simulink library "speedgoatlib_bce"  (R2024b)
settings: Solver=VariableStepAuto  StartTime=0.0  StopTime=10.0  RelTol=1e-3
undefined symbols (not defined in the file): BCE12, BCE_Set_init, Cell_1, Cell_10, Cell_11, Cell_12, Cell_2, Cell_3, Cell_4, Cell_5, Cell_6, Cell_7, Cell_8, Cell_9, Device_01, FIU12, sg_bce, TSE04
libraries: slrealtimeethercatlib x292, simulink x92, slrealtimeutilitieslib x24
(part 3 of 4)

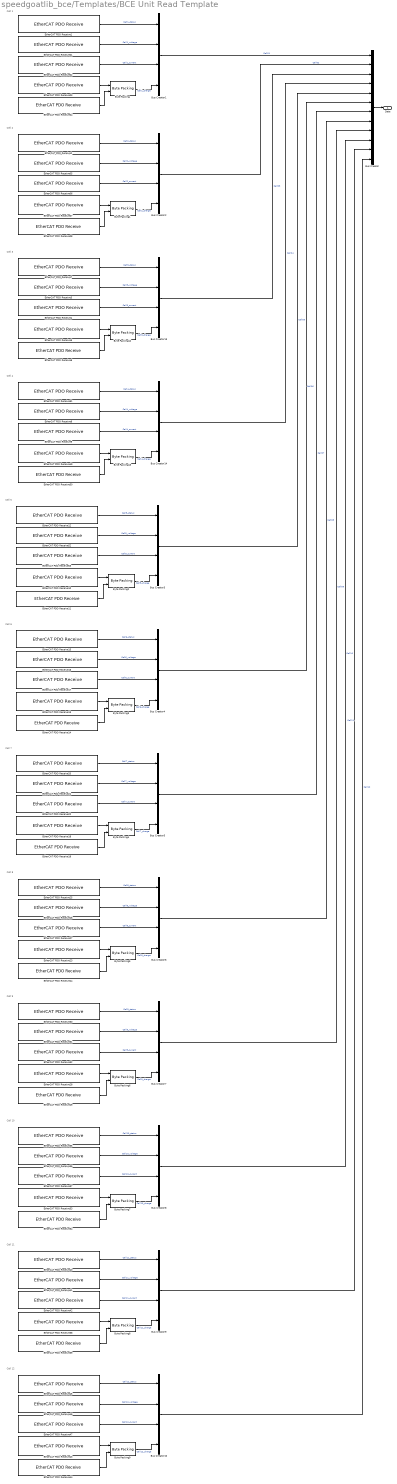
== system speedgoatlib_bce/Templates/BCE Unit Read Template  ==
  note: Cell 1
  note: Cell 9
  note: Cell 10
  note: Cell 4
  note: Cell 5
  note: Cell 3
  note: Cell 11
  note: Cell 12
  note: Cell 8
  note: Cell 6
  note: Cell 2
  note: Cell 7
  Bus Creator : BusCreator  Inputs=12  OutDataTypeStr=Bus: BCE_Get
      settings: InheritFromInputs=off
  Bus Creator{1..10,13..14} (12 alike) : BusCreator  Inputs=4  OutDataTypeStr=Bus: Cell_Get
      settings: InheritFromInputs=off
  Byte Packing{,1..9,12..13} (12 alike) : slrealtimeutilitieslib/Byte Packing  MaskPackedDataType=uint64  MaskUnpackedDataTypes={'uint32','uint32'}  MaskAlignment=1
  EtherCAT PDO Receive01 : slrealtimeethercatlib/EtherCAT PDO Receive  Priority=2  sig_name=Device_01 (BCE12-0505).Tx_Cell_01.voltage  sig_offset=16  sig_type=single  type_size=32  sig_dim=1  device_id=0  sample_time=0.000000
  EtherCAT PDO Receive02 : slrealtimeethercatlib/EtherCAT PDO Receive  Priority=2  sig_name=Device_01 (BCE12-0505).Tx_Cell_01.current  sig_offset=48  sig_type=single  type_size=32  sig_dim=1  device_id=0  sample_time=0.000000
  EtherCAT PDO Receive03 : slrealtimeethercatlib/EtherCAT PDO Receive  Priority=2  sig_name=Device_01 (BCE12-0505).Tx_Cell_01.chargeMSB  sig_offset=80  sig_type=uint32  type_size=32  sig_dim=1  device_id=0  sample_time=0.000000
  EtherCAT PDO Receive04 : slrealtimeethercatlib/EtherCAT PDO Receive  Priority=2  sig_name=Device_01 (BCE12-0505).Tx_Cell_01.chargeLSB  sig_offset=112  sig_type=uint32  type_size=32  sig_dim=1  device_id=0  sample_time=0.000000
  EtherCAT PDO Receive05 : slrealtimeethercatlib/EtherCAT PDO Receive  Priority=2  sig_name=Device_01 (BCE12-0505).Tx_Cell_02.voltage  sig_offset=160  sig_type=single  type_size=32  sig_dim=1  device_id=0  sample_time=0.000000
  EtherCAT PDO Receive06 : slrealtimeethercatlib/EtherCAT PDO Receive  Priority=2  sig_name=Device_01 (BCE12-0505).Tx_Cell_02.current  sig_offset=192  sig_type=single  type_size=32  sig_dim=1  device_id=0  sample_time=0.000000
  EtherCAT PDO Receive07 : slrealtimeethercatlib/EtherCAT PDO Receive  Priority=2  sig_name=Device_01 (BCE12-0505).Tx_Cell_02.chargeMSB  sig_offset=224  sig_type=uint32  type_size=32  sig_dim=1  device_id=0  sample_time=0.000000
  EtherCAT PDO Receive08 : slrealtimeethercatlib/EtherCAT PDO Receive  Priority=2  sig_name=Device_01 (BCE12-0505).Tx_Cell_02.chargeLSB  sig_offset=256  sig_type=uint32  type_size=32  sig_dim=1  device_id=0  sample_time=0.000000
  EtherCAT PDO Receive1 : slrealtimeethercatlib/EtherCAT PDO Receive  Priority=2  sig_name=Device_01 (BCE12-0505).Tx_Cell_01.status  sig_offset=0  sig_type=uint16  type_size=16  sig_dim=1  device_id=0  sample_time=0.000000
  EtherCAT PDO Receive10 : slrealtimeethercatlib/EtherCAT PDO Receive  Priority=2  sig_name=Device_01 (BCE12-0505).Tx_Cell_05.chargeMSB  sig_offset=656  sig_type=uint32  type_size=32  sig_dim=1  device_id=0  sample_time=0.000000
  EtherCAT PDO Receive11 : slrealtimeethercatlib/EtherCAT PDO Receive  Priority=2  sig_name=Device_01 (BCE12-0505).Tx_Cell_05.chargeLSB  sig_offset=688  sig_type=uint32  type_size=32  sig_dim=1  device_id=0  sample_time=0.000000
  EtherCAT PDO Receive12 : slrealtimeethercatlib/EtherCAT PDO Receive  Priority=2  sig_name=Device_01 (BCE12-0505).Tx_Cell_05.status  sig_offset=576  sig_type=uint16  type_size=16  sig_dim=1  device_id=0  sample_time=0.000000
  EtherCAT PDO Receive13 : slrealtimeethercatlib/EtherCAT PDO Receive  Priority=2  sig_name=Device_01 (BCE12-0505).Tx_Cell_06.chargeMSB  sig_offset=800  sig_type=uint32  type_size=32  sig_dim=1  device_id=0  sample_time=0.000000
  EtherCAT PDO Receive14 : slrealtimeethercatlib/EtherCAT PDO Receive  Priority=2  sig_name=Device_01 (BCE12-0505).Tx_Cell_06.chargeLSB  sig_offset=832  sig_type=uint32  type_size=32  sig_dim=1  device_id=0  sample_time=0.000000
  EtherCAT PDO Receive15 : slrealtimeethercatlib/EtherCAT PDO Receive  Priority=2  sig_name=Device_01 (BCE12-0505).Tx_Cell_06.status  sig_offset=720  sig_type=uint16  type_size=16  sig_dim=1  device_id=0  sample_time=0.000000
  EtherCAT PDO Receive16 : slrealtimeethercatlib/EtherCAT PDO Receive  Priority=2  sig_name=Device_01 (BCE12-0505).Tx_Cell_06.voltage  sig_offset=736  sig_type=single  type_size=32  sig_dim=1  device_id=0  sample_time=0.000000
  EtherCAT PDO Receive17 : slrealtimeethercatlib/EtherCAT PDO Receive  Priority=2  sig_name=Device_01 (BCE12-0505).Tx_Cell_06.current  sig_offset=768  sig_type=single  type_size=32  sig_dim=1  device_id=0  sample_time=0.000000
  EtherCAT PDO Receive18 : slrealtimeethercatlib/EtherCAT PDO Receive  Priority=2  sig_name=Device_01 (BCE12-0505).Tx_Cell_07.chargeMSB  sig_offset=944  sig_type=uint32  type_size=32  sig_dim=1  device_id=0  sample_time=0.000000
  EtherCAT PDO Receive19 : slrealtimeethercatlib/EtherCAT PDO Receive  Priority=2  sig_name=Device_01 (BCE12-0505).Tx_Cell_07.chargeLSB  sig_offset=976  sig_type=uint32  type_size=32  sig_dim=1  device_id=0  sample_time=0.000000
  EtherCAT PDO Receive2 : slrealtimeethercatlib/EtherCAT PDO Receive  Priority=2  sig_name=Device_01 (BCE12-0505).Tx_Cell_02.status  sig_offset=144  sig_type=uint16  type_size=16  sig_dim=1  device_id=0  sample_time=0.000000
  EtherCAT PDO Receive20 : slrealtimeethercatlib/EtherCAT PDO Receive  Priority=2  sig_name=Device_01 (BCE12-0505).Tx_Cell_07.status  sig_offset=864  sig_type=uint16  type_size=16  sig_dim=1  device_id=0  sample_time=0.000000
  EtherCAT PDO Receive21 : slrealtimeethercatlib/EtherCAT PDO Receive  Priority=2  sig_name=Device_01 (BCE12-0505).Tx_Cell_07.voltage  sig_offset=880  sig_type=single  type_size=32  sig_dim=1  device_id=0  sample_time=0.000000
  EtherCAT PDO Receive22 : slrealtimeethercatlib/EtherCAT PDO Receive  Priority=2  sig_name=Device_01 (BCE12-0505).Tx_Cell_07.current  sig_offset=912  sig_type=single  type_size=32  sig_dim=1  device_id=0  sample_time=0.000000
  EtherCAT PDO Receive23 : slrealtimeethercatlib/EtherCAT PDO Receive  Priority=2  sig_name=Device_01 (BCE12-0505).Tx_Cell_08.chargeMSB  sig_offset=1088  sig_type=uint32  type_size=32  sig_dim=1  device_id=0  sample_time=0.000000
  EtherCAT PDO Receive24 : slrealtimeethercatlib/EtherCAT PDO Receive  Priority=2  sig_name=Device_01 (BCE12-0505).Tx_Cell_08.chargeLSB  sig_offset=1120  sig_type=uint32  type_size=32  sig_dim=1  device_id=0  sample_time=0.000000
  EtherCAT PDO Receive25 : slrealtimeethercatlib/EtherCAT PDO Receive  Priority=2  sig_name=Device_01 (BCE12-0505).Tx_Cell_08.status  sig_offset=1008  sig_type=uint16  type_size=16  sig_dim=1  device_id=0  sample_time=0.000000
  EtherCAT PDO Receive26 : slrealtimeethercatlib/EtherCAT PDO Receive  Priority=2  sig_name=Device_01 (BCE12-0505).Tx_Cell_08.voltage  sig_offset=1024  sig_type=single  type_size=32  sig_dim=1  device_id=0  sample_time=0.000000
  EtherCAT PDO Receive27 : slrealtimeethercatlib/EtherCAT PDO Receive  Priority=2  sig_name=Device_01 (BCE12-0505).Tx_Cell_08.current  sig_offset=1056  sig_type=single  type_size=32  sig_dim=1  device_id=0  sample_time=0.000000
  EtherCAT PDO Receive28 : slrealtimeethercatlib/EtherCAT PDO Receive  Priority=2  sig_name=Device_01 (BCE12-0505).Tx_Cell_09.chargeMSB  sig_offset=1232  sig_type=uint32  type_size=32  sig_dim=1  device_id=0  sample_time=0.000000
  EtherCAT PDO Receive29 : slrealtimeethercatlib/EtherCAT PDO Receive  Priority=2  sig_name=Device_01 (BCE12-0505).Tx_Cell_09.chargeLSB  sig_offset=1264  sig_type=uint32  type_size=32  sig_dim=1  device_id=0  sample_time=0.000000
  EtherCAT PDO Receive3 : slrealtimeethercatlib/EtherCAT PDO Receive  Priority=2  sig_name=Device_01 (BCE12-0505).Tx_Cell_03.voltage  sig_offset=304  sig_type=single  type_size=32  sig_dim=1  device_id=0  sample_time=0.000000
  EtherCAT PDO Receive30 : slrealtimeethercatlib/EtherCAT PDO Receive  Priority=2  sig_name=Device_01 (BCE12-0505).Tx_Cell_09.status  sig_offset=1152  sig_type=uint16  type_size=16  sig_dim=1  device_id=0  sample_time=0.000000
  EtherCAT PDO Receive31 : slrealtimeethercatlib/EtherCAT PDO Receive  Priority=2  sig_name=Device_01 (BCE12-0505).Tx_Cell_09.voltage  sig_offset=1168  sig_type=single  type_size=32  sig_dim=1  device_id=0  sample_time=0.000000
  EtherCAT PDO Receive32 : slrealtimeethercatlib/EtherCAT PDO Receive  Priority=2  sig_name=Device_01 (BCE12-0505).Tx_Cell_09.current  sig_offset=1200  sig_type=single  type_size=32  sig_dim=1  device_id=0  sample_time=0.000000
  EtherCAT PDO Receive33 : slrealtimeethercatlib/EtherCAT PDO Receive  Priority=2  sig_name=Device_01 (BCE12-0505).Tx_Cell_10.chargeMSB  sig_offset=1376  sig_type=uint32  type_size=32  sig_dim=1  device_id=0  sample_time=0.000000
  EtherCAT PDO Receive34 : slrealtimeethercatlib/EtherCAT PDO Receive  Priority=2  sig_name=Device_01 (BCE12-0505).Tx_Cell_10.chargeLSB  sig_offset=1408  sig_type=uint32  type_size=32  sig_dim=1  device_id=0  sample_time=0.000000
  EtherCAT PDO Receive35 : slrealtimeethercatlib/EtherCAT PDO Receive  Priority=2  sig_name=Device_01 (BCE12-0505).Tx_Cell_10.status  sig_offset=1296  sig_type=uint16  type_size=16  sig_dim=1  device_id=0  sample_time=0.000000
  EtherCAT PDO Receive36 : slrealtimeethercatlib/EtherCAT PDO Receive  Priority=2  sig_name=Device_01 (BCE12-0505).Tx_Cell_10.voltage  sig_offset=1312  sig_type=single  type_size=32  sig_dim=1  device_id=0  sample_time=0.000000
  EtherCAT PDO Receive37 : slrealtimeethercatlib/EtherCAT PDO Receive  Priority=2  sig_name=Device_01 (BCE12-0505).Tx_Cell_10.current  sig_offset=1344  sig_type=single  type_size=32  sig_dim=1  device_id=0  sample_time=0.000000
  EtherCAT PDO Receive38 : slrealtimeethercatlib/EtherCAT PDO Receive  Priority=2  sig_name=Device_01 (BCE12-0505).Tx_Cell_11.chargeMSB  sig_offset=1520  sig_type=uint32  type_size=32  sig_dim=1  device_id=0  sample_time=0.000000
  EtherCAT PDO Receive39 : slrealtimeethercatlib/EtherCAT PDO Receive  Priority=2  sig_name=Device_01 (BCE12-0505).Tx_Cell_11.chargeLSB  sig_offset=1552  sig_type=uint32  type_size=32  sig_dim=1  device_id=0  sample_time=0.000000
  EtherCAT PDO Receive4 : slrealtimeethercatlib/EtherCAT PDO Receive  Priority=2  sig_name=Device_01 (BCE12-0505).Tx_Cell_03.current  sig_offset=336  sig_type=single  type_size=32  sig_dim=1  device_id=0  sample_time=0.000000
  EtherCAT PDO Receive40 : slrealtimeethercatlib/EtherCAT PDO Receive  Priority=2  sig_name=Device_01 (BCE12-0505).Tx_Cell_11.status  sig_offset=1440  sig_type=uint16  type_size=16  sig_dim=1  device_id=0  sample_time=0.000000
  EtherCAT PDO Receive41 : slrealtimeethercatlib/EtherCAT PDO Receive  Priority=2  sig_name=Device_01 (BCE12-0505).Tx_Cell_11.voltage  sig_offset=1456  sig_type=single  type_size=32  sig_dim=1  device_id=0  sample_time=0.000000
  EtherCAT PDO Receive42 : slrealtimeethercatlib/EtherCAT PDO Receive  Priority=2  sig_name=Device_01 (BCE12-0505).Tx_Cell_11.current  sig_offset=1488  sig_type=single  type_size=32  sig_dim=1  device_id=0  sample_time=0.000000
  EtherCAT PDO Receive43 : slrealtimeethercatlib/EtherCAT PDO Receive  Priority=2  sig_name=Device_01 (BCE12-0505).Tx_Cell_12.chargeMSB  sig_offset=1664  sig_type=uint32  type_size=32  sig_dim=1  device_id=0  sample_time=0.000000
  EtherCAT PDO Receive44 : slrealtimeethercatlib/EtherCAT PDO Receive  Priority=2  sig_name=Device_01 (BCE12-0505).Tx_Cell_12.chargeLSB  sig_offset=1696  sig_type=uint32  type_size=32  sig_dim=1  device_id=0  sample_time=0.000000
  EtherCAT PDO Receive45 : slrealtimeethercatlib/EtherCAT PDO Receive  Priority=2  sig_name=Device_01 (BCE12-0505).Tx_Cell_12.status  sig_offset=1584  sig_type=uint16  type_size=16  sig_dim=1  device_id=0  sample_time=0.000000
  EtherCAT PDO Receive46 : slrealtimeethercatlib/EtherCAT PDO Receive  Priority=2  sig_name=Device_01 (BCE12-0505).Tx_Cell_12.voltage  sig_offset=1600  sig_type=single  type_size=32  sig_dim=1  device_id=0  sample_time=0.000000
  EtherCAT PDO Receive47 : slrealtimeethercatlib/EtherCAT PDO Receive  Priority=2  sig_name=Device_01 (BCE12-0505).Tx_Cell_12.current  sig_offset=1632  sig_type=single  type_size=32  sig_dim=1  device_id=0  sample_time=0.000000
  EtherCAT PDO Receive49 : slrealtimeethercatlib/EtherCAT PDO Receive  Priority=2  sig_name=Device_01 (BCE12-0505).Tx_Cell_04.chargeMSB  sig_offset=512  sig_type=uint32  type_size=32  sig_dim=1  device_id=0  sample_time=0.000000
  EtherCAT PDO Receive5 : slrealtimeethercatlib/EtherCAT PDO Receive  Priority=2  sig_name=Device_01 (BCE12-0505).Tx_Cell_03.chargeMSB  sig_offset=368  sig_type=uint32  type_size=32  sig_dim=1  device_id=0  sample_time=0.000000
  EtherCAT PDO Receive50 : slrealtimeethercatlib/EtherCAT PDO Receive  Priority=2  sig_name=Device_01 (BCE12-0505).Tx_Cell_04.chargeLSB  sig_offset=544  sig_type=uint32  type_size=32  sig_dim=1  device_id=0  sample_time=0.000000
  EtherCAT PDO Receive51 : slrealtimeethercatlib/EtherCAT PDO Receive  Priority=2  sig_name=Device_01 (BCE12-0505).Tx_Cell_04.status  sig_offset=432  sig_type=uint16  type_size=16  sig_dim=1  device_id=0  sample_time=0.000000
  EtherCAT PDO Receive52 : slrealtimeethercatlib/EtherCAT PDO Receive  Priority=2  sig_name=Device_01 (BCE12-0505).Tx_Cell_05.voltage  sig_offset=592  sig_type=single  type_size=32  sig_dim=1  device_id=0  sample_time=0.000000
  EtherCAT PDO Receive53 : slrealtimeethercatlib/EtherCAT PDO Receive  Priority=2  sig_name=Device_01 (BCE12-0505).Tx_Cell_05.current  sig_offset=624  sig_type=single  type_size=32  sig_dim=1  device_id=0  sample_time=0.000000
  EtherCAT PDO Receive6 : slrealtimeethercatlib/EtherCAT PDO Receive  Priority=2  sig_name=Device_01 (BCE12-0505).Tx_Cell_03.chargeLSB  sig_offset=400  sig_type=uint32  type_size=32  sig_dim=1  device_id=0  sample_time=0.000000
  EtherCAT PDO Receive7 : slrealtimeethercatlib/EtherCAT PDO Receive  Priority=2  sig_name=Device_01 (BCE12-0505).Tx_Cell_03.status  sig_offset=288  sig_type=uint16  type_size=16  sig_dim=1  device_id=0  sample_time=0.000000
  EtherCAT PDO Receive8 : slrealtimeethercatlib/EtherCAT PDO Receive  Priority=2  sig_name=Device_01 (BCE12-0505).Tx_Cell_04.voltage  sig_offset=448  sig_type=single  type_size=32  sig_dim=1  device_id=0  sample_time=0.000000
  EtherCAT PDO Receive9 : slrealtimeethercatlib/EtherCAT PDO Receive  Priority=2  sig_name=Device_01 (BCE12-0505).Tx_Cell_04.current  sig_offset=480  sig_type=single  type_size=32  sig_dim=1  device_id=0  sample_time=0.000000
  Data : Outport  OutDataTypeStr=Bus: BCE_Get
  wires:
  EtherCAT PDO Receive08/1 -> Byte Packing1/2
  EtherCAT PDO Receive03/1 -> Byte Packing/1
  Bus Creator/1 -> Data/1
  EtherCAT PDO Receive2/1 -> Bus Creator2/1  "Cell2_status"
  EtherCAT PDO Receive34/1 -> Byte Packing7/2
  EtherCAT PDO Receive02/1 -> Bus Creator1/3  "Cell1_current"
  EtherCAT PDO Receive42/1 -> Bus Creator9/3  "Cell11_current"
  EtherCAT PDO Receive20/1 -> Bus Creator5/1  "Cell7_status"
  EtherCAT PDO Receive10/1 -> Byte Packing2/1
  EtherCAT PDO Receive47/1 -> Bus Creator10/3  "Cell12_current"
  EtherCAT PDO Receive07/1 -> Byte Packing1/1
  EtherCAT PDO Receive36/1 -> Bus Creator8/2  "Cell10_voltage"
  Bus Creator1/1 -> Bus Creator/1  "Cell01"
  Byte Packing5/1 -> Bus Creator6/4  "Cell8_charge"
  Byte Packing9/1 -> Bus Creator10/4  "Cell12_charge"
  EtherCAT PDO Receive22/1 -> Bus Creator5/3  "Cell7_current"
  Bus Creator3/1 -> Bus Creator/5  "Cell05"
  EtherCAT PDO Receive50/1 -> Byte Packing13/2
  EtherCAT PDO Receive38/1 -> Byte Packing8/1
  Byte Packing/1 -> Bus Creator1/4  "Cell1_charge"
  Byte Packing12/1 -> Bus Creator13/4  "Cell3_charge"
  EtherCAT PDO Receive31/1 -> Bus Creator7/2  "Cell9_voltage"
  EtherCAT PDO Receive25/1 -> Bus Creator6/1  "Cell8_status"
  EtherCAT PDO Receive06/1 -> Bus Creator2/3  "Cell2_current"
  EtherCAT PDO Receive05/1 -> Bus Creator2/2  "Cell2_voltage"
  EtherCAT PDO Receive51/1 -> Bus Creator14/1  "Cell4_status"
  EtherCAT PDO Receive16/1 -> Bus Creator4/2  "Cell6_voltage"
  EtherCAT PDO Receive13/1 -> Byte Packing3/1
  Byte Packing3/1 -> Bus Creator4/4  "Cell6_charge"
  EtherCAT PDO Receive28/1 -> Byte Packing6/1
  Bus Creator8/1 -> Bus Creator/10  "Cell10"
  Bus Creator10/1 -> Bus Creator/12  "Cell12"
  Byte Packing1/1 -> Bus Creator2/4  "Cell2_charge"
  Byte Packing8/1 -> Bus Creator9/4  "Cell11_charge"
  Bus Creator5/1 -> Bus Creator/7  "Cell07"
  Bus Creator2/1 -> Bus Creator/2  "Cell02"
  EtherCAT PDO Receive24/1 -> Byte Packing5/2
  EtherCAT PDO Receive19/1 -> Byte Packing4/2
  EtherCAT PDO Receive49/1 -> Byte Packing13/1
  EtherCAT PDO Receive14/1 -> Byte Packing3/2
  EtherCAT PDO Receive8/1 -> Bus Creator14/2  "Cell4_voltage"
  EtherCAT PDO Receive37/1 -> Bus Creator8/3  "Cell10_current"
  EtherCAT PDO Receive23/1 -> Byte Packing5/1
  EtherCAT PDO Receive45/1 -> Bus Creator10/1  "Cell12_status"
  EtherCAT PDO Receive44/1 -> Byte Packing9/2
  EtherCAT PDO Receive43/1 -> Byte Packing9/1
  Bus Creator9/1 -> Bus Creator/11  "Cell11"
  EtherCAT PDO Receive9/1 -> Bus Creator14/3  "Cell4_current"
  EtherCAT PDO Receive17/1 -> Bus Creator4/3  "Cell6_current"
  EtherCAT PDO Receive6/1 -> Byte Packing12/2
  EtherCAT PDO Receive46/1 -> Bus Creator10/2  "Cell12_voltage"
  EtherCAT PDO Receive3/1 -> Bus Creator13/2  "Cell3_voltage"
  EtherCAT PDO Receive5/1 -> Byte Packing12/1
  EtherCAT PDO Receive41/1 -> Bus Creator9/2  "Cell11_voltage"
  EtherCAT PDO Receive32/1 -> Bus Creator7/3  "Cell9_current"
  EtherCAT PDO Receive27/1 -> Bus Creator6/3  "Cell8_current"
  EtherCAT PDO Receive29/1 -> Byte Packing6/2
  EtherCAT PDO Receive35/1 -> Bus Creator8/1  "Cell10_status"
  EtherCAT PDO Receive01/1 -> Bus Creator1/2  "Cell1_voltage"
  Byte Packing7/1 -> Bus Creator8/4  "Cell10_charge"
  Bus Creator13/1 -> Bus Creator/3  "Cell03"
  EtherCAT PDO Receive4/1 -> Bus Creator13/3  "Cell3_current"
  EtherCAT PDO Receive30/1 -> Bus Creator7/1  "Cell9_status"
  Bus Creator6/1 -> Bus Creator/8  "Cell08"
  Bus Creator4/1 -> Bus Creator/6  "Cell06"
  EtherCAT PDO Receive7/1 -> Bus Creator13/1  "Cell3_status"
  Byte Packing6/1 -> Bus Creator7/4  "Cell9_charge"
  Byte Packing4/1 -> Bus Creator5/4  "Cell7_charge"
  Byte Packing2/1 -> Bus Creator3/4  "Cell5_charge"
  EtherCAT PDO Receive12/1 -> Bus Creator3/1  "Cell5_status"
  EtherCAT PDO Receive33/1 -> Byte Packing7/1
  EtherCAT PDO Receive26/1 -> Bus Creator6/2  "Cell8_voltage"
  EtherCAT PDO Receive11/1 -> Byte Packing2/2
  EtherCAT PDO Receive15/1 -> Bus Creator4/1  "Cell6_status"
  EtherCAT PDO Receive52/1 -> Bus Creator3/2  "Cell5_voltage"
  EtherCAT PDO Receive21/1 -> Bus Creator5/2  "Cell7_voltage"
  Bus Creator14/1 -> Bus Creator/4  "Cell04"
  Byte Packing13/1 -> Bus Creator14/4  "Cell4_charge"
  EtherCAT PDO Receive18/1 -> Byte Packing4/1
  EtherCAT PDO Receive39/1 -> Byte Packing8/2
  EtherCAT PDO Receive40/1 -> Bus Creator9/1  "Cell11_status"
  EtherCAT PDO Receive1/1 -> Bus Creator1/1  "Cell1_status"
  Bus Creator7/1 -> Bus Creator/9  "Cell09"
  EtherCAT PDO Receive53/1 -> Bus Creator3/3  "Cell5_current"
  EtherCAT PDO Receive04/1 -> Byte Packing/2

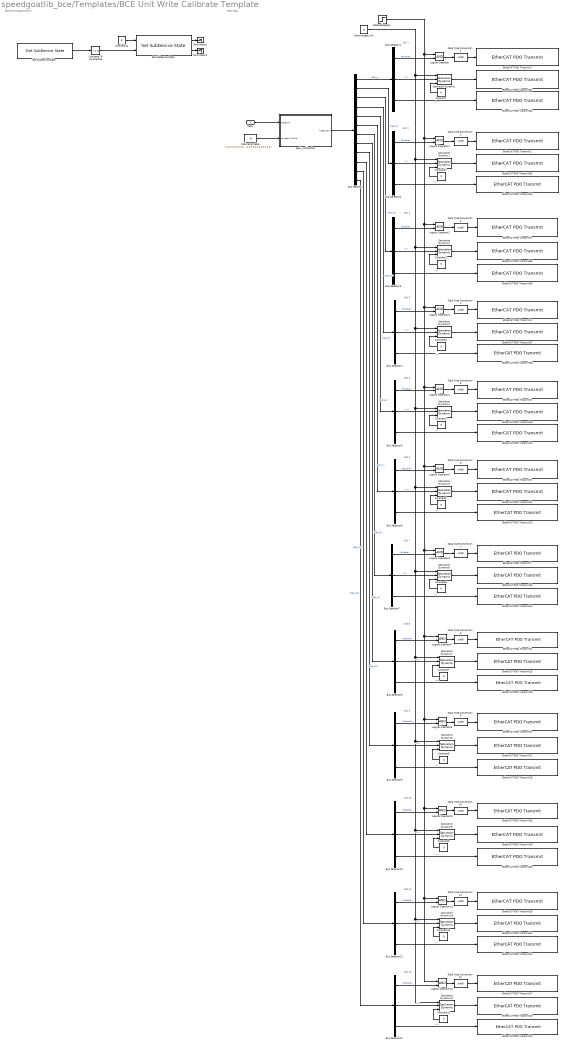
== system speedgoatlib_bce/Templates/BCE Unit Write Calibrate Template  ==
  note: Cell 2
  note: Cell 12
  note: Cell 11
  note: Cell 6
  note: Cell 10
  note: Cell 3
  note: Cell 5
  note: PDO Data
  note: Cell 7
  note: Cell 1
  note: Cell 9
  note: Cell 8
  note: Cell 4
  note: EtherCAT State Control
  Data : Inport  OutDataTypeStr=Bus: BCE_Set
  BceVoltageLimit : Constant  Value=6
  Bus Selector : BusSelector  OutputSignals=Cell_1,Cell_2,Cell_3,Cell_4,Cell_5,Cell_6,Cell_7,Cell_8,Cell_9,Cell_10,Cell_11,Cell_12
  Bus Selector{1..12} (12 alike) : BusSelector  OutputSignals=Enable,V,I
  CalibrationTable : Constant  Value=[1 0 1 0;1 0 1 0;1 0 1 0;1 0 1 0;1 0 1 0;1 0 1 0;1 0 1 0;1 0 1 0;1 0 1 0;1 0 1 0;1 0 1 0;1 0 1 0]
  CellEnableDelay : Step  Time=2  SampleTime=0
  Compare To Constant25 : simulink/Logic and Bit Operations/Compare To Constant  relop=~=  const=8  OutDataTypeStr=boolean
  Constant{,1..11} (12 alike) : Constant  Value=0
  Constant12 : Constant  Value=8  OutDataTypeStr=int32
  Data Type Conversion{1..12} (12 alike) : DataTypeConversion  OutDataTypeStr=uint8  SaturateOnIntegerOverflow=off  RndMeth=Floor
  EtherCAT PDO Transmit01 : slrealtimeethercatlib/EtherCAT PDO Transmit  Priority=3  sig_name=Device_01 (BCE12-0605).Rx_Cell_01.setVoltage  sig_offset=8  sig_type=single  type_size=32  sig_dim=1  device_id=0  sample_time=0.001000
  EtherCAT PDO Transmit02 : slrealtimeethercatlib/EtherCAT PDO Transmit  Priority=3  sig_name=Device_01 (BCE12-0605).Rx_Cell_01.setCurrent  sig_offset=40  sig_type=single  type_size=32  sig_dim=1  device_id=0  sample_time=0.001000
  EtherCAT PDO Transmit03 : slrealtimeethercatlib/EtherCAT PDO Transmit  Priority=3  sig_name=Device_01 (BCE12-0605).Rx_Cell_02.setVoltage  sig_offset=80  sig_type=single  type_size=32  sig_dim=1  device_id=0  sample_time=0.001000
  EtherCAT PDO Transmit04 : slrealtimeethercatlib/EtherCAT PDO Transmit  Priority=3  sig_name=Device_01 (BCE12-0605).Rx_Cell_02.setCurrent  sig_offset=112  sig_type=single  type_size=32  sig_dim=1  device_id=0  sample_time=0.001000
  EtherCAT PDO Transmit05 : slrealtimeethercatlib/EtherCAT PDO Transmit  Priority=3  sig_name=Device_01 (BCE12-0605).Rx_Cell_03.setVoltage  sig_offset=152  sig_type=single  type_size=32  sig_dim=1  device_id=0  sample_time=0.001000
  EtherCAT PDO Transmit06 : slrealtimeethercatlib/EtherCAT PDO Transmit  Priority=3  sig_name=Device_01 (BCE12-0605).Rx_Cell_03.setCurrent  sig_offset=184  sig_type=single  type_size=32  sig_dim=1  device_id=0  sample_time=0.001000
  EtherCAT PDO Transmit07 : slrealtimeethercatlib/EtherCAT PDO Transmit  Priority=3  sig_name=Device_01 (BCE12-0605).Rx_Cell_04.setVoltage  sig_offset=224  sig_type=single  type_size=32  sig_dim=1  device_id=0  sample_time=0.001000
  EtherCAT PDO Transmit08 : slrealtimeethercatlib/EtherCAT PDO Transmit  Priority=3  sig_name=Device_01 (BCE12-0605).Rx_Cell_04.setCurrent  sig_offset=256  sig_type=single  type_size=32  sig_dim=1  device_id=0  sample_time=0.001000
  EtherCAT PDO Transmit09 : slrealtimeethercatlib/EtherCAT PDO Transmit  Priority=3  sig_name=Device_01 (BCE12-0605).Rx_Cell_05.setVoltage  sig_offset=296  sig_type=single  type_size=32  sig_dim=1  device_id=0  sample_time=0.001000
  EtherCAT PDO Transmit1 : slrealtimeethercatlib/EtherCAT PDO Transmit  Priority=3  sig_name=Device_01 (BCE12-0605).Rx_Cell_01.enableCell  sig_offset=0  sig_type=uint8  type_size=8  sig_dim=1  device_id=0  sample_time=0.001000
  EtherCAT PDO Transmit10 : slrealtimeethercatlib/EtherCAT PDO Transmit  Priority=3  sig_name=Device_01 (BCE12-0605).Rx_Cell_05.setCurrent  sig_offset=328  sig_type=single  type_size=32  sig_dim=1  device_id=0  sample_time=0.001000
  EtherCAT PDO Transmit11 : slrealtimeethercatlib/EtherCAT PDO Transmit  Priority=3  sig_name=Device_01 (BCE12-0605).Rx_Cell_06.setVoltage  sig_offset=368  sig_type=single  type_size=32  sig_dim=1  device_id=0  sample_time=0.001000
  EtherCAT PDO Transmit12 : slrealtimeethercatlib/EtherCAT PDO Transmit  Priority=3  sig_name=Device_01 (BCE12-0605).Rx_Cell_06.setCurrent  sig_offset=400  sig_type=single  type_size=32  sig_dim=1  device_id=0  sample_time=0.001000
  EtherCAT PDO Transmit13 : slrealtimeethercatlib/EtherCAT PDO Transmit  Priority=3  sig_name=Device_01 (BCE12-0605).Rx_Cell_07.setVoltage  sig_offset=440  sig_type=single  type_size=32  sig_dim=1  device_id=0  sample_time=0.001000
  EtherCAT PDO Transmit14 : slrealtimeethercatlib/EtherCAT PDO Transmit  Priority=3  sig_name=Device_01 (BCE12-0605).Rx_Cell_07.setCurrent  sig_offset=472  sig_type=single  type_size=32  sig_dim=1  device_id=0  sample_time=0.001000
  EtherCAT PDO Transmit15 : slrealtimeethercatlib/EtherCAT PDO Transmit  Priority=3  sig_name=Device_01 (BCE12-0605).Rx_Cell_08.setVoltage  sig_offset=512  sig_type=single  type_size=32  sig_dim=1  device_id=0  sample_time=0.001000
  EtherCAT PDO Transmit16 : slrealtimeethercatlib/EtherCAT PDO Transmit  Priority=3  sig_name=Device_01 (BCE12-0605).Rx_Cell_08.setCurrent  sig_offset=544  sig_type=single  type_size=32  sig_dim=1  device_id=0  sample_time=0.001000
  EtherCAT PDO Transmit17 : slrealtimeethercatlib/EtherCAT PDO Transmit  Priority=3  sig_name=Device_01 (BCE12-0605).Rx_Cell_09.setVoltage  sig_offset=584  sig_type=single  type_size=32  sig_dim=1  device_id=0  sample_time=0.001000
  EtherCAT PDO Transmit18 : slrealtimeethercatlib/EtherCAT PDO Transmit  Priority=3  sig_name=Device_01 (BCE12-0605).Rx_Cell_09.setCurrent  sig_offset=616  sig_type=single  type_size=32  sig_dim=1  device_id=0  sample_time=0.001000
  EtherCAT PDO Transmit19 : slrealtimeethercatlib/EtherCAT PDO Transmit  Priority=3  sig_name=Device_01 (BCE12-0605).Rx_Cell_10.setVoltage  sig_offset=656  sig_type=single  type_size=32  sig_dim=1  device_id=0  sample_time=0.001000
  EtherCAT PDO Transmit2 : slrealtimeethercatlib/EtherCAT PDO Transmit  Priority=3  sig_name=Device_01 (BCE12-0605).Rx_Cell_02.enableCell  sig_offset=72  sig_type=uint8  type_size=8  sig_dim=1  device_id=0  sample_time=0.001000
  EtherCAT PDO Transmit20 : slrealtimeethercatlib/EtherCAT PDO Transmit  Priority=3  sig_name=Device_01 (BCE12-0605).Rx_Cell_10.setCurrent  sig_offset=688  sig_type=single  type_size=32  sig_dim=1  device_id=0  sample_time=0.001000
  EtherCAT PDO Transmit21 : slrealtimeethercatlib/EtherCAT PDO Transmit  Priority=3  sig_name=Device_01 (BCE12-0605).Rx_Cell_11.setVoltage  sig_offset=728  sig_type=single  type_size=32  sig_dim=1  device_id=0  sample_time=0.001000
  EtherCAT PDO Transmit22 : slrealtimeethercatlib/EtherCAT PDO Transmit  Priority=3  sig_name=Device_01 (BCE12-0605).Rx_Cell_11.setCurrent  sig_offset=760  sig_type=single  type_size=32  sig_dim=1  device_id=0  sample_time=0.001000
  EtherCAT PDO Transmit23 : slrealtimeethercatlib/EtherCAT PDO Transmit  Priority=3  sig_name=Device_01 (BCE12-0605).Rx_Cell_12.setVoltage  sig_offset=800  sig_type=single  type_size=32  sig_dim=1  device_id=0  sample_time=0.001000
  EtherCAT PDO Transmit24 : slrealtimeethercatlib/EtherCAT PDO Transmit  Priority=3  sig_name=Device_01 (BCE12-0605).Rx_Cell_12.setCurrent  sig_offset=832  sig_type=single  type_size=32  sig_dim=1  device_id=0  sample_time=0.001000
  EtherCAT PDO Transmit25 : slrealtimeethercatlib/EtherCAT PDO Transmit  Priority=3  sig_name=Device_01 (BCE12-0605).Rx_Cell_10.enableCell  sig_offset=648  sig_type=uint8  type_size=8  sig_dim=1  device_id=0  sample_time=0.001000
  EtherCAT PDO Transmit26 : slrealtimeethercatlib/EtherCAT PDO Transmit  Priority=3  sig_name=Device_01 (BCE12-0605).Rx_Cell_11.enableCell  sig_offset=720  sig_type=uint8  type_size=8  sig_dim=1  device_id=0  sample_time=0.001000
  EtherCAT PDO Transmit27 : slrealtimeethercatlib/EtherCAT PDO Transmit  Priority=3  sig_name=Device_01 (BCE12-0605).Rx_Cell_12.enableCell  sig_offset=792  sig_type=uint8  type_size=8  sig_dim=1  device_id=0  sample_time=0.001000
  EtherCAT PDO Transmit3 : slrealtimeethercatlib/EtherCAT PDO Transmit  Priority=3  sig_name=Device_01 (BCE12-0605).Rx_Cell_03.enableCell  sig_offset=144  sig_type=uint8  type_size=8  sig_dim=1  device_id=0  sample_time=0.001000
  EtherCAT PDO Transmit4 : slrealtimeethercatlib/EtherCAT PDO Transmit  Priority=3  sig_name=Device_01 (BCE12-0605).Rx_Cell_04.enableCell  sig_offset=216  sig_type=uint8  type_size=8  sig_dim=1  device_id=0  sample_time=0.001000
  EtherCAT PDO Transmit5 : slrealtimeethercatlib/EtherCAT PDO Transmit  Priority=3  sig_name=Device_01 (BCE12-0605).Rx_Cell_05.enableCell  sig_offset=288  sig_type=uint8  type_size=8  sig_dim=1  device_id=0  sample_time=0.001000
  EtherCAT PDO Transmit6 : slrealtimeethercatlib/EtherCAT PDO Transmit  Priority=3  sig_name=Device_01 (BCE12-0605).Rx_Cell_06.enableCell  sig_offset=360  sig_type=uint8  type_size=8  sig_dim=1  device_id=0  sample_time=0.001000
  EtherCAT PDO Transmit7 : slrealtimeethercatlib/EtherCAT PDO Transmit  Priority=3  sig_name=Device_01 (BCE12-0605).Rx_Cell_07.enableCell  sig_offset=432  sig_type=uint8  type_size=8  sig_dim=1  device_id=0  sample_time=0.001000
  EtherCAT PDO Transmit8 : slrealtimeethercatlib/EtherCAT PDO Transmit  Priority=3  sig_name=Device_01 (BCE12-0605).Rx_Cell_08.enableCell  sig_offset=504  sig_type=uint8  type_size=8  sig_dim=1  device_id=0  sample_time=0.001000
  EtherCAT PDO Transmit9 : slrealtimeethercatlib/EtherCAT PDO Transmit  Priority=3  sig_name=Device_01 (BCE12-0605).Rx_Cell_09.enableCell  sig_offset=576  sig_type=uint8  type_size=8  sig_dim=1  device_id=0  sample_time=0.001000
  Get SubDevice State : slrealtimeethercatlib/Get SubDevice State  device_id=0  sample_time=1  subdevice_addr=0  selected_subdevice=Term 1 (EK1100)  timeout=500  subdevice_found=0
  Logical Operator{,1..11} (12 alike) : Logic  AllPortsSameDT=off  OutDataTypeStr=boolean
  Saturation Dynamic{,1..11} (12 alike) : simulink/Discontinuities/Saturation Dynamic  OutMin=[]  OutMax=[]  OutDataTypeStr=Inherit: Same as second input  OutDataType=fixdt(1, 16)  OutScaling=2^-10  DoSatur=off
  Set SubDevice State : slrealtimeethercatlib/Set SubDevice State  device_id=0  sample_time=1  subdevice_addr=0  selected_subdevice=Term 1 (EK1100)  subdevice_found=0
  Terminator1 : Terminator
  Terminator2 : Terminator
  apply_calibration : Subsystem
  wires:
  apply_calibration/1(bceBusOut) -> Bus Selector/1
  CalibrationTable/1 -> apply_calibration/2(correctionTable)
  Data/1 -> apply_calibration/1(bceBusIn)
  Data Type Conversion8/1 -> EtherCAT PDO Transmit8/1
  Bus Selector9/2 -> Saturation Dynamic8/2  "<V>"
  Bus Selector12/2 -> Saturation Dynamic11/2  "<V>"
  Bus Selector2/2 -> Saturation Dynamic1/2  "<V>"
  Bus Selector/7 -> Bus Selector7/1  "<Cell_7>"
  Bus Selector11/2 -> Saturation Dynamic10/2  "<V>"
  Bus Selector/1 -> Bus Selector1/1  "<Cell_1>"
  Bus Selector8/3 -> EtherCAT PDO Transmit16/1  "<I>"
  Bus Selector/3 -> Bus Selector3/1  "<Cell_3>"
  Bus Selector1/2 -> Saturation Dynamic/2  "<V>"
  Bus Selector/2 -> Bus Selector2/1  "<Cell_2>"
  Bus Selector/6 -> Bus Selector6/1  "<Cell_6>"
  Data Type Conversion2/1 -> EtherCAT PDO Transmit2/1
  Bus Selector7/2 -> Saturation Dynamic6/2  "<V>"
  Bus Selector7/3 -> EtherCAT PDO Transmit14/1  "<I>"
  Bus Selector/9 -> Bus Selector9/1  "<Cell_9>"
  Data Type Conversion4/1 -> EtherCAT PDO Transmit4/1
  Data Type Conversion6/1 -> EtherCAT PDO Transmit6/1
  Data Type Conversion9/1 -> EtherCAT PDO Transmit9/1
  Data Type Conversion5/1 -> EtherCAT PDO Transmit5/1
  Data Type Conversion12/1 -> EtherCAT PDO Transmit27/1
  Data Type Conversion10/1 -> EtherCAT PDO Transmit25/1
  Data Type Conversion1/1 -> EtherCAT PDO Transmit1/1
  Bus Selector4/3 -> EtherCAT PDO Transmit08/1  "<I>"
  Bus Selector/12 -> Bus Selector12/1  "<Cell_12>"
  Bus Selector3/3 -> EtherCAT PDO Transmit06/1  "<I>"
  Bus Selector6/2 -> Saturation Dynamic5/2  "<V>"
  Bus Selector4/2 -> Saturation Dynamic3/2  "<V>"
  Data Type Conversion3/1 -> EtherCAT PDO Transmit3/1
  Bus Selector1/3 -> EtherCAT PDO Transmit02/1  "<I>"
  Bus Selector/10 -> Bus Selector10/1  "<Cell_10>"
  Bus Selector/5 -> Bus Selector5/1  "<Cell_5>"
  Bus Selector12/3 -> EtherCAT PDO Transmit24/1  "<I>"
  Bus Selector10/2 -> Saturation Dynamic9/2  "<V>"
  Bus Selector2/3 -> EtherCAT PDO Transmit04/1  "<I>"
  Bus Selector3/2 -> Saturation Dynamic2/2  "<V>"
  Bus Selector/11 -> Bus Selector11/1  "<Cell_11>"
  Bus Selector10/3 -> EtherCAT PDO Transmit20/1  "<I>"
  Bus Selector5/3 -> EtherCAT PDO Transmit10/1  "<I>"
  Data Type Conversion11/1 -> EtherCAT PDO Transmit26/1
  Bus Selector5/2 -> Saturation Dynamic4/2  "<V>"
  Bus Selector8/2 -> Saturation Dynamic7/2  "<V>"
  Bus Selector/8 -> Bus Selector8/1  "<Cell_8>"
  Bus Selector9/3 -> EtherCAT PDO Transmit18/1  "<I>"
  Bus Selector11/3 -> EtherCAT PDO Transmit22/1  "<I>"
  Data Type Conversion7/1 -> EtherCAT PDO Transmit7/1
  Bus Selector/4 -> Bus Selector4/1  "<Cell_4>"
  Bus Selector6/3 -> EtherCAT PDO Transmit12/1  "<I>"
  Saturation Dynamic/1 -> EtherCAT PDO Transmit01/1
  Constant/1 -> Saturation Dynamic/3
  BceVoltageLimit/1 -> Saturation Dynamic/1, Saturation Dynamic11/1, Saturation Dynamic10/1, Saturation Dynamic9/1, Saturation Dynamic8/1, Saturation Dynamic7/1, Saturation Dynamic6/1, Saturation Dynamic5/1, Saturation Dynamic4/1, Saturation Dynamic3/1, Saturation Dynamic2/1, Saturation Dynamic1/1
  Constant1/1 -> Saturation Dynamic1/3
  Saturation Dynamic1/1 -> EtherCAT PDO Transmit03/1
  Constant2/1 -> Saturation Dynamic2/3
  Saturation Dynamic2/1 -> EtherCAT PDO Transmit05/1
  Constant3/1 -> Saturation Dynamic3/3
  Saturation Dynamic3/1 -> EtherCAT PDO Transmit07/1
  Constant4/1 -> Saturation Dynamic4/3
  Saturation Dynamic4/1 -> EtherCAT PDO Transmit09/1
  Constant5/1 -> Saturation Dynamic5/3
  Saturation Dynamic5/1 -> EtherCAT PDO Transmit11/1
  Constant6/1 -> Saturation Dynamic6/3
  Saturation Dynamic6/1 -> EtherCAT PDO Transmit13/1
  Constant7/1 -> Saturation Dynamic7/3
  Saturation Dynamic7/1 -> EtherCAT PDO Transmit15/1
  Constant8/1 -> Saturation Dynamic8/3
  Saturation Dynamic8/1 -> EtherCAT PDO Transmit17/1
  Constant9/1 -> Saturation Dynamic9/3
  Saturation Dynamic9/1 -> EtherCAT PDO Transmit19/1
  Constant10/1 -> Saturation Dynamic10/3
  Saturation Dynamic10/1 -> EtherCAT PDO Transmit21/1
  Constant11/1 -> Saturation Dynamic11/3
  Saturation Dynamic11/1 -> EtherCAT PDO Transmit23/1
  Get SubDevice State/1 -> Compare To Constant25/1
  Set SubDevice State/2 -> Terminator2/1
  Set SubDevice State/1 -> Terminator1/1
  Compare To Constant25/1 -> Set SubDevice State/2
  Constant12/1 -> Set SubDevice State/1
  CellEnableDelay/1 -> Logical Operator11/1, Logical Operator10/1, Logical Operator9/1, Logical Operator8/1, Logical Operator7/1, Logical Operator6/1, Logical Operator5/1, Logical Operator4/1, Logical Operator3/1, Logical Operator2/1, Logical Operator1/1, Logical Operator/1
  Bus Selector1/1 -> Logical Operator/2  "<Enable>"
  Logical Operator/1 -> Data Type Conversion1/1
  Bus Selector2/1 -> Logical Operator1/2  "<Enable>"
  Logical Operator1/1 -> Data Type Conversion2/1
  Bus Selector3/1 -> Logical Operator2/2  "<Enable>"
  Logical Operator2/1 -> Data Type Conversion3/1
  Bus Selector4/1 -> Logical Operator3/2  "<Enable>"
  Logical Operator3/1 -> Data Type Conversion4/1
  Bus Selector5/1 -> Logical Operator4/2  "<Enable>"
  Logical Operator4/1 -> Data Type Conversion5/1
  Bus Selector6/1 -> Logical Operator5/2  "<Enable>"
  Logical Operator5/1 -> Data Type Conversion6/1
  Bus Selector7/1 -> Logical Operator6/2  "<Enable>"
  Logical Operator6/1 -> Data Type Conversion7/1
  Bus Selector8/1 -> Logical Operator7/2  "<Enable>"
  Logical Operator7/1 -> Data Type Conversion8/1
  Bus Selector9/1 -> Logical Operator8/2  "<Enable>"
  Logical Operator8/1 -> Data Type Conversion9/1
  Bus Selector10/1 -> Logical Operator9/2  "<Enable>"
  Logical Operator9/1 -> Data Type Conversion10/1
  Bus Selector11/1 -> Logical Operator10/2  "<Enable>"
  Logical Operator10/1 -> Data Type Conversion11/1
  Bus Selector12/1 -> Logical Operator11/2  "<Enable>"
  Logical Operator11/1 -> Data Type Conversion12/1
